simulink model "sgMdl_IO104_AnalogDigitalLoopback"  (R2024b)
settings: Solver=FixedStepAuto  StartTime=0.0  StopTime=inf  RelTol=1e-3  EnableMultiTasking=on
undefined symbols (not defined in the file): Ended, Single
libraries: speedgoatlib_IO104 x5
Description:
  | IO104 - Analog and Digital Loopback
settings Model: ModifiedByFormat=Speedgoat  SimulationMode=external  ExtModeTrigDuration=100000  Creator=Speedgoat  LastModifiedBy=Speedgoat
settings SolverCC: ConcurrentTasks=on  AlgebraicLoopSolver=TrustRegion  PositivePriorityOrder=on
settings DataIOCC: LimitDataPoints=on  SaveFormat=Array  SignalLoggingSaveFormat=ModelDataLogs  ReturnWorkspaceOutputs=off
settings OptimizationCC: BlockReduction=off  OptimizeBlockIOStorage=off  BufferReuse=off  GlobalBufferReuse=off  ExpressionFolding=off  ExpressionDepthLimit=2147483647  LocalBlockOutputs=off
settings DebuggingCC: UnderspecifiedInitializationDetection=Classic  MergeDetectMultiDrivingBlocksExec=none  SolverPrmCheckMsg=warning  TasksWithSamePriorityMsg=none  FcnCallInpInsideContextMsg=warning  StateNameClashWarn=warning  SFUnexpectedBacktrackingDiag=warning  SFNoUnconditionalDefaultTransitionDiag=warning  SFExecutionAtInitializationDiag=none  ArithmeticOperatorsInVariantConditions=warning
settings HardwareCC: ProdBitPerLong=64  ProdLongLongMode=on  ProdHWDeviceType=Intel->x86-64 (Linux 64)
settings ModelReferenceCC: EnableRefExpFcnMdlSchedulingChecks=on  PropagateSignalLabelsOutOfModel=off
settings SFSimCC: SimUseLocalCustomCode=off  CustomCodeUndefinedFunction=UseInterfaceOnly
settings RTWCC: Description=Speedgoat Real-Time Target Machine  SystemTargetFile=speedgoat.tlc  TemplateMakefile=slrealtime_default_tmf  RTWUseLocalCustomCode=off  Toolchain=Simulink Real-Time Toolchain  BuildConfiguration=Faster Runs  TargetLang=C++  GPUComputeCapability=3.5  DLArmComputeVersion=19.05
settings CodeAppCC: StateflowObjectComments=on
settings SimulinkRealTimeTargetCC: SubcomponentCodeInterfacePackaging=Reusable function  InstructionSetFMA=off  LogToMDFFile=off  SLRTFileLogMaxRuns=10  UseGCCFastMath=on
settings ConfigComp: CovMetricSettings=dw  CovSaveCumulativeToWorkspaceVar=on  CovSaveSingleToWorkspaceVar=on  CovExternalEMLEnable=off  CovSFcnEnable=off  CovBoundaryAbsTol=1.0e-5

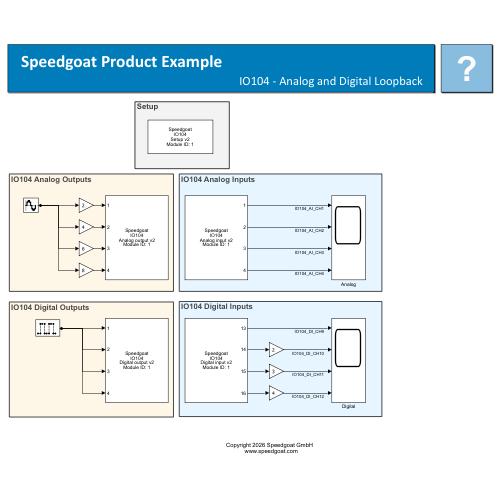
[thumbnail: Simulink's stored preview of the top-level diagram]
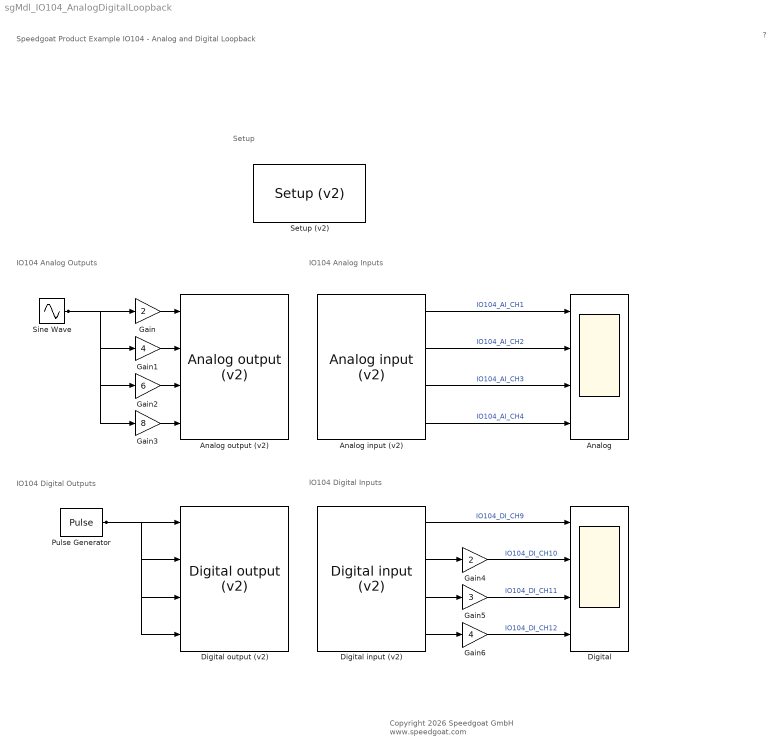
== system sgMdl_IO104_AnalogDigitalLoopback ==
  note: IO104 Analog Outputs
  note: IO104 Analog Inputs
  note: IO104 Digital Outputs
  note: IO104 Digital Inputs
  note: Setup
  note: Speedgoat Product Example
      | IO104 - Analog and Digital Loopback
  note: ?
  note: Copyright 2026 Speedgoat GmbH
      |  www.speedgoat.com
  Analog : Scope  NumInputPorts=4
  "Analog input (v2) " : speedgoatlib_IO104/Analog input (v2)   parModuleId=1  parTs=1e-3  parPciSlot=-1  parAdChannels=[1,2,3,4]  parAdChannelsSorted=[1,2,3,4]  parAdRange1=+-10V  parAdRange2=+-10V  parAdCoupling=Single-Ended  parAdFrameSize=1  parAdUseTrigger=off  parAdClockInitiator=Initiator  parAdSampleTime=1.000000000e-03  parTriggerInitiator=Initiator  parTriggerRate=-1.000000000e+00
      settings: SourceProductName=Simulink Real-Time: Speedgoat Library
  "Analog output (v2) " : speedgoatlib_IO104/Analog output (v2)   parModuleId=1  parTs=1e-3  parPciSlot=-1  parDaSimultaneous=on  parDaChannels=[1,2,3,4]  parDaChannelsSorted=[1,2,3,4]  parDaInitValue=[0,0,0,0]  parDaReset=[1,1,1,1]  parDaRange=+-10V  parDaFrameSize=1  parDaUseTrigger=off  parDaClockInitiator=Initiator  parDaSampleTime=1.000000000e-03  parTriggerInitiator=Initiator  parTriggerRate=-1.000000000e+00  parAdBlockPresent=1
      settings: SourceProductName=Simulink Real-Time: Speedgoat Library
  Digital : Scope  NumInputPorts=4
  "Digital input (v2) " : speedgoatlib_IO104/Digital input (v2)   parModuleId=1  parTs=1e-3  parPciSlot=-1  parDiChannels=[9,10,11,12]
      settings: SourceProductName=Simulink Real-Time: Speedgoat Library
  "Digital output (v2) " : speedgoatlib_IO104/Digital output (v2)   parModuleId=1  parTs=1e-3  parDoChannels=[1,2,3,4]  parDoInitValues=[0,0,0,0]  parDoReset=[1,1,1,1]  parPciSlot=-1
      settings: SourceProductName=Simulink Real-Time: Speedgoat Library
  Gain : Gain  Gain=2
  Gain1 : Gain  Gain=4
  Gain2 : Gain  Gain=6
  Gain3 : Gain  Gain=8
  Gain4 : Gain  Gain=2
  Gain5 : Gain  Gain=3
  Gain6 : Gain  Gain=4
  Pulse Generator : DiscretePulseGenerator  Period=20  PulseWidth=10  SampleTime=1e-3
  "Setup (v2) " : speedgoatlib_IO104/Setup (v2)   parPciSlot=-1  parModuleId=1  parTriggerInitiator=Initiator  parTriggerRate=1e-3  parCalibrate=on  parAdChannels=[1, 2, 3, 4]  parAdRange1=+-10V  parAdRange2=+-10V  parAdCoupling=Single-Ended  parAdUseTrigger=off  parAdFrameSize=1  parAdClockInitiator=Initiator  parAdSampleTime=1e-3  parDaSimultaneous=on  parDaChannels=[1:4]  parDaChannelsSorted=[1,2,3,4]  parDaInitValue=[0]  parDaReset=[1]  parDaRange=+-10V  parDaUseTrigger=off  parDaFrameSize=1  parDaClockInitiator=Initiator  parDaSampleTime=1e-3  parDioByte0Dir=Outputs  parDioByte1Dir=Inputs  parDoChannels=[1:4]  parDoInitValues=[0]  parDoReset=[1]  parDiChannels=[9, 10, 11, 12]
      settings: SourceProductName=Simulink Real-Time: Speedgoat Library
  Sine Wave : Sin  Frequency=2*pi*50  SampleTime=1e-3
  wires:
  Gain/1 -> "Analog output (v2) "/1
  Gain1/1 -> "Analog output (v2) "/2
  Gain2/1 -> "Analog output (v2) "/3
  Gain3/1 -> "Analog output (v2) "/4
  Sine Wave/1 -> Gain3/1, Gain2/1, Gain1/1, Gain/1
  "Digital input (v2) "/2 -> Gain4/1
  "Digital input (v2) "/3 -> Gain5/1
  "Digital input (v2) "/4 -> Gain6/1
  Pulse Generator/1 -> "Digital output (v2) "/1, "Digital output (v2) "/4, "Digital output (v2) "/3, "Digital output (v2) "/2
  "Analog input (v2) "/1 -> Analog/1  "IO104_AI_CH1"
  "Analog input (v2) "/2 -> Analog/2  "IO104_AI_CH2"
  "Analog input (v2) "/3 -> Analog/3  "IO104_AI_CH3"
  "Analog input (v2) "/4 -> Analog/4  "IO104_AI_CH4"
  "Digital input (v2) "/1 -> Digital/1  "IO104_DI_CH9"
  Gain4/1 -> Digital/2  "IO104_DI_CH10"
  Gain5/1 -> Digital/3  "IO104_DI_CH11"
  Gain6/1 -> Digital/4  "IO104_DI_CH12"
